simulink library "lib_vehicle_nodiv"  (Simulink 7.7)
settings: Solver=ode45  SolverMode=SingleTasking  StartTime=0.0  StopTime=10.0  RelTol=1e-3
undefined symbols (not defined in the file): M, T_veh, v0, v_max
settings Model: Creator=yt59680  LastModifiedBy=lfeng

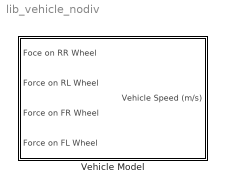
== system lib_vehicle_nodiv ==
  Vehicle Model : Subsystem  TreatAsAtomicUnit=on
      settings: MinAlgLoopOccurrences=on

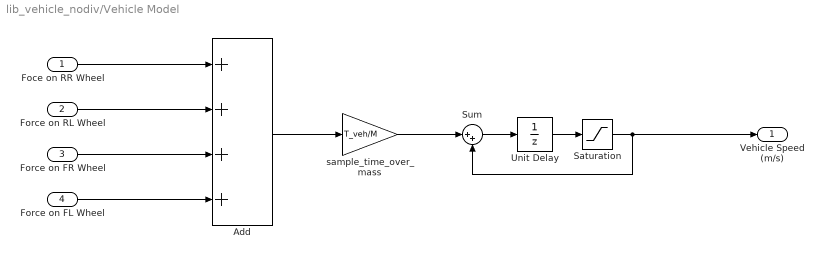
== system lib_vehicle_nodiv/Vehicle Model ==
  Foce on RR Wheel : Inport
  Force on RL Wheel : Inport  Port=2
  Force on FR Wheel : Inport  Port=3
  Force on FL Wheel : Inport  Port=4
  Add : Sum  Inputs=++++
  Saturation : Saturate  UpperLimit=v_max  LowerLimit=0
  Sum : Sum  Inputs=|++
  Unit Delay : UnitDelay  X0=v0  SampleTime=-1
  sample_time_over_mass : Gain  Gain=T_veh/M
  Vehicle Speed (m/s) : Outport
  wires:
  Sum/1 -> Unit Delay/1
  Unit Delay/1 -> Saturation/1
  Saturation/1 -> Sum/2, Vehicle Speed (m/s)/1
  Foce on RR Wheel/1 -> Add/1
  Force on RL Wheel/1 -> Add/2
  Force on FR Wheel/1 -> Add/3
  Force on FL Wheel/1 -> Add/4
  Add/1 -> sample_time_over_mass/1
  sample_time_over_mass/1 -> Sum/1
